simulink model "STEVE_ver28"  (R2022a)
settings: Solver=VariableStepAuto  StartTime=0.0  StopTime=Stop_Time  FixedStep=0.000001  RelTol=1e-5
values from neighbouring files (symbols this model uses):
  Bed_ave_OD = (1+Bed_ins_OD)/2    (= 1.667)    [STEVE_initialization.m]    (also in STEVE_running.m = (1+Bed_ins_OD)/2; STEVE_v4_C1Demo_2023_Nominal.m)
  Bed_ins_OD = 2.334    [STEVE_initialization.m]    (also in STEVE_v4_C1Demo_2023_Nominal.m)
  Bed_thickness = 0.049    [STEVE_initialization.m]    (also in STEVE_v4_C1Demo_2023_Nominal.m)
  Belimo_Cv = 16    [STEVE_initialization.m]    (also in STEVE_v4_C1Demo_2023_Nominal.m)
  flow_rate = 8    [STEVE_initialization.m]    (also in STEVE_v4_C1Demo_2023_Nominal.m)
  Heat_ads = 40000    [STEVE_initialization.m]    (also in STEVE_v4_C1Demo_2023_Nominal.m)
  Heater_output = 85.3    [STEVE_initialization.m]    (also in STEVE_v4_C1Demo_2023_Nominal.m)
  L = 0.508    [STEVE_initialization.m]    (also in STEVE_v4_C1Demo_2023_Nominal.m)
  L_inch = L*39.3701    (= 20.0000108)    [STEVE_initialization.m]    (also in STEVE_v4_C1Demo_2023_Nominal.m)
  max_temp = 200+273.15    (= 473.15)    [STEVE_initialization.m]    (also in STEVE_v4_C1Demo_2023_Nominal.m)
  mesh_size = 15    [STEVE_initialization.m]    (also in STEVE_v4_C1Demo_2023_Nominal.m)
  Pipe_ave_HD = (pipe_HD+0.5)/2    (= 0.465)    [STEVE_initialization.m]    (also in STEVE_running.m = (pipe_HD+0.5)/2; STEVE_v4_C1Demo_2023_Nominal.m)
  pipe_HD = 0.43    [STEVE_initialization.m]    (also in STEVE_v4_C1Demo_2023_Nominal.m)
  Ramp_rate = 0.0833    [STEVE_initialization.m]    (also in STEVE_v4_C1Demo_2023_Nominal.m)
  room_pressure = 13.3    [STEVE_initialization.m]    (also in STEVE_v4_C1Demo_2023_Nominal.m)
  t_Total = Adsorption_time + FlowStop_time + Valve_close_Time + Select_valve_close_Time + Pump_down_time + Desorption_time + SelectValve_open_Time + Valve_open_Time    (= 9635)    [STEVE_initialization.m]    (also in STEVE_running.m = Adsorption_time + FlowStop_time + Valve_close_Time + Select_; STEVE_v4_C1Demo_2023_Nominal.m)
libraries: fl_lib x229, nesl_utility x75, slpidlib x2
(part 2 of 5)

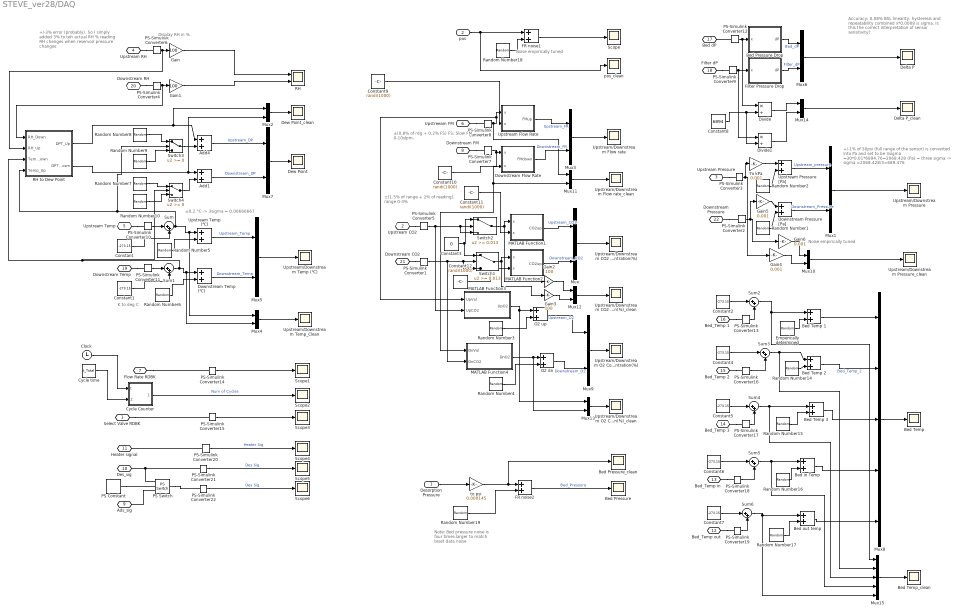
== system STEVE_ver28/DAQ ==
  note: Note: Bed pressure noise is four times larger to match teset data noise
  note: ±(1.5% of range + 2% of reading), range 0-3%
  note: ±0.2 °C -> 3sigma = 0.06666667
  note: ±(0.8% of rdg + 0.2% FS)
      | FS: Slow FM 0-10slpm,
  note: Accuracy: 0.08% BSL linearity, hysteresis and repeatability combined
      |
      | x*0.0008 is sigma. Is this the correct interpretation of sensor sensitivity?
  note: +/-1% of 30psi (full range of the sensor) is converted into Pa and set to be 3sigma
      | =30*0.01*6894.76=2068.428 (Pa) = three sigma  -> sigma =2068.428/3=689.476
  note: +/-3% error (probably). So I simply added 3% to teh actual RH % reading
      | RH chenges when reservoir pressure changes
  note: Display RH in %
  note: K to deg C
  note: Noise empirically tuned
  note: Noise empirically tuned
  Desorption Pressure : Inport
  pos : Inport  Port=2
  Add1 : Sum
  Add4 : Sum
  Bed Pressure : Scope
  Bed Pressure Drop : MATLAB Function  TreatAsAtomicUnit=on
  Bed Pressure_clean : Scope
  Bed Temp : Scope
  Bed Temp 1 : Sum
  Bed Temp 2 : Sum
  Bed Temp 3 : Sum
  Bed Temp_clean : Scope
  Bed in Temp : Sum
  Bed out temp : Sum
  Clock : Clock
  Constant{,1..2,4..7} (7 alike) : Constant  Value=-273.15
  Constant{9..12} (4 alike) : Constant  Value=randi(1000)
  Constant3 : Constant  Value=0
  Constant8 : Constant  Value=6894
  Cycle Counter : MATLAB Function  TreatAsAtomicUnit=on
  Cycle time : Constant  Value=t_Total
  Delta P : Scope
  Delta P_clean : Scope
  Dew Point : Scope
  Dew Point_clean : Scope
  Divide : Product  Inputs=*/
  Divide1 : Product  Inputs=*/
  Downstream Pressure [Pa] : Sum
  Downstream Temp (℃) : Sum
  Downstream Flow Rate : MATLAB Function  TreatAsAtomicUnit=on
  Emperically determined : RandomNumber  Variance=0.0197^2  Seed=randi(1000)  SampleTime=1  VectorParams1D=off
  FR noise1 : Sum
  FR noise2 : Sum
  Filter Pressure Drop : MATLAB Function  TreatAsAtomicUnit=on
  Gain{,1..3} (4 alike) : Gain  Gain=100
  Gain4 : Gain  Gain=0.001
  Gain5 : Gain  Gain=0.001
  Gain6 : Gain  Gain=0.001
  MATLAB Function1 : MATLAB Function  TreatAsAtomicUnit=on
  MATLAB Function2 : MATLAB Function  TreatAsAtomicUnit=on
  MATLAB Function3 : MATLAB Function  TreatAsAtomicUnit=on
  MATLAB Function4 : MATLAB Function  TreatAsAtomicUnit=on
  Mux{,1..7,9..14} (14 alike) : Mux  Inputs=2
  Mux15 : Mux  Inputs=5
  Mux8 : Mux  Inputs=5
  O2 dn : Sum
  O2 up : Sum
  PS Constant : fl_lib/Physical Signals/Sources/PS Constant  constant=0
      settings: SourceProductBaseCode=PW,SS,VE
  PS Switch : fl_lib/Physical Signals/Nonlinear Operators/PS Switch  Threshold=1
      settings: SourceProductBaseCode=PW,SS,VE  InternalSimscapePortConfiguration="{\"Bottom\":[],\"Left\":[{\"id\":\"I1\",\"label\":\"\",\"type\":\"input\"},{\"id\":\"I2\",\"label\":\"\",\"type\":\"input\"},{\"id\":\"I3\",\"label\":\"\",\"type\":\"input\"}],\"Right\":[{\"id\":\"O\",\"label\":\"\",\"type\":\"output\"}],\"Top\":[]}"
  PS-Simulink Converter{1,4..6,14..15,20..22} (9 alike) : nesl_utility/PS-Simulink Converter  PhysicalDomain=network_engine_domain  SubClassName=ps_output  LeftPortType=input  RightPortType=output  PseudoPeriodic=off  Frequencies=[]  VectorFormat=1-D array  Unit=inherit  AffineConversion=off
      settings: SourceProductBaseCode=SS,PW,VE
  PS-Simulink Converter{10..11,13,16..19} (7 alike) : nesl_utility/PS-Simulink Converter  PhysicalDomain=network_engine_domain  SubClassName=ps_output  LeftPortType=input  RightPortType=output  PseudoPeriodic=off  Frequencies=[]  VectorFormat=1-D array  Unit=K  AffineConversion=off
      settings: SourceProductBaseCode=SS,PW,VE
  PS-Simulink Converter{2..3,9,12} (4 alike) : nesl_utility/PS-Simulink Converter  PhysicalDomain=network_engine_domain  SubClassName=ps_output  LeftPortType=input  RightPortType=output  PseudoPeriodic=off  Frequencies=[]  VectorFormat=1-D array  Unit=Pa  AffineConversion=off
      settings: SourceProductBaseCode=SS,PW,VE
  PS-Simulink Converter7 : nesl_utility/PS-Simulink Converter  PhysicalDomain=network_engine_domain  SubClassName=ps_output  LeftPortType=input  RightPortType=output  PseudoPeriodic=off  Frequencies=[]  VectorFormat=1-D array  Unit=lpm  AffineConversion=off
      settings: SourceProductBaseCode=SS,PW,VE
  PS-Simulink Converter8 : nesl_utility/PS-Simulink Converter  PhysicalDomain=network_engine_domain  SubClassName=ps_output  LeftPortType=input  RightPortType=output  PseudoPeriodic=off  Frequencies=[]  VectorFormat=1-D array  Unit=lpm  AffineConversion=off
      settings: SourceProductBaseCode=SS,PW,VE
  RH : Scope  NumInputPorts=2
  RH to Dew Point : MATLAB Function  TreatAsAtomicUnit=on
  Random Number1 : RandomNumber  Variance=0.0068  Seed=randi(1000)  SampleTime=1  VectorParams1D=off
  Random Number10 : RandomNumber  Variance=(4/3)^2  Seed=randi(1000)  SampleTime=1  VectorParams1D=off
  Random Number{14..17} (4 alike) : RandomNumber  Variance=0.0197^2  Seed=randi(1000)  SampleTime=1  VectorParams1D=off
  Random Number18 : RandomNumber  Variance=0.0542  Seed=randi(1000)  SampleTime=1  VectorParams1D=off
  Random Number19 : RandomNumber  Variance=0.0326^2  Seed=randi(1000)  SampleTime=1  VectorParams1D=off
  Random Number2 : RandomNumber  Variance=0.0068  Seed=randi(1000)  SampleTime=1  VectorParams1D=off
  Random Number3 : RandomNumber  Variance=0.0175^2  Seed=randi(1000)  SampleTime=1  VectorParams1D=off
  Random Number4 : RandomNumber  Variance=0.0175^2  Seed=randi(1000)  SampleTime=1  VectorParams1D=off
  Random Number5 : RandomNumber  Variance=(0.06666667/3)^2  Seed=randi(1000)  SampleTime=1  VectorParams1D=off
  Random Number6 : RandomNumber  Variance=(0.06666667/3)^2  Seed=randi(1000)  SampleTime=1  VectorParams1D=off
  Random Number7 : RandomNumber  Variance=(2/3)^2  Seed=randi(1000)  SampleTime=1  VectorParams1D=off
  Random Number8 : RandomNumber  Variance=(2/3)^2  Seed=randi(1000)  SampleTime=1  VectorParams1D=off
  Random Number9 : RandomNumber  Variance=(4/3)^2  Seed=randi(1000)  SampleTime=1  VectorParams1D=off
  Scope{,1..6} (7 alike) : Scope
  Sum{,1..6} (7 alike) : Sum  Inputs=|++
  Switch1 : Switch  Threshold=0.013  SaturateOnIntegerOverflow=off  InputSameDT=off
  Switch2 : Switch  Threshold=0.013  SaturateOnIntegerOverflow=off  InputSameDT=off
  Switch3 : Switch  SaturateOnIntegerOverflow=off  InputSameDT=off
  Switch4 : Switch  SaturateOnIntegerOverflow=off  InputSameDT=off
  To kPa : Gain  Gain=0.001
  Upstream Pressure [Pa] : Sum
  Upstream Temp (℃) : Sum
  Upstream Flow Rate : MATLAB Function  TreatAsAtomicUnit=on
  Upstream/Downstream CO2 Concentration(%) : Scope
  Upstream/Downstream CO2 Concentration(%)_clean : Scope
  Upstream/Downstream Flow rate : Scope
  Upstream/Downstream O2 Concentration(%) : Scope
  Upstream/Downstream O2 Concentration(%)_clean : Scope
  Upstream/Downstream Pressure : Scope
  Upstream/Downstream Pressure_clean : Scope
  Upstream/Downstream Temp (℃) : Scope
  Upstream/Downstream Flow rate_clean : Scope
  Upstream/Downstream Temp_Clean : Scope
  pos_clean : Scope
  to psi : Gain  Gain=0.000145
  Select Valve RDBK : PMIOPort  Side=Left
  Upstream CO2 : PMIOPort  Port=2  Side=Left
  Upstream Pressure : PMIOPort  Port=3  Side=Left
  Upstream RH : PMIOPort  Port=4  Side=Left
  Upstream Temp : PMIOPort  Port=5  Side=Left
  Upstreeam FM : PMIOPort  Port=6  Side=Left
  Flow Rate RDBK : PMIOPort  Port=7  Side=Left
  Downstream FM : PMIOPort  Port=8  Side=Left
  Ads_sig : PMIOPort  Port=9  Side=Left
  Des_sig : PMIOPort  Port=10  Side=Left
  Heater signal : PMIOPort  Port=11  Side=Right
  Bed_Temp out : PMIOPort  Port=12  Side=Right
  Bed_Temp in : PMIOPort  Port=13  Side=Right
  Bed_Temp 3 : PMIOPort  Port=14  Side=Right
  Bed_Temp 2 : PMIOPort  Port=15  Side=Right
  Bed_Temp 1 : PMIOPort  Port=16  Side=Right
  Bed dP : PMIOPort  Port=17  Side=Right
  Filter dP : PMIOPort  Port=18  Side=Right
  Downstream Temp : PMIOPort  Port=19  Side=Right
  Downstream RH : PMIOPort  Port=20  Side=Right
  Downstream CO2 : PMIOPort  Port=21  Side=Right
  Downstream Pressure : PMIOPort  Port=22  Side=Right
  wires:
  Mux1/1 -> Upstream/Downstream Pressure/1
  Mux3/1 -> Upstream/Downstream Flow rate/1
  Mux5/1 -> Upstream/Downstream Temp (℃)/1
  Random Number1/1 -> Downstream Pressure [Pa]/2
  Random Number2/1 -> Upstream Pressure [Pa]/2
  PS-Simulink Converter6/1 -> RH to Dew Point/2(RH_Up), Gain/1
  PS-Simulink Converter4/1 -> RH to Dew Point/1(RH_Down), Gain1/1
  PS-Simulink Converter8/1 -> Mux11/1, MATLAB Function3/1(UpVol), Upstream Flow Rate/1(x)
  PS-Simulink Converter7/1 -> Mux11/2, MATLAB Function4/1(DnVol), Downstream Flow Rate/1(x)
  Downstream Flow Rate/1(FMdown) -> Mux3/2  "Downstream_FR"
  Upstream Flow Rate/1(FMup) -> Mux3/1  "Upstream_FR"
  Random Number5/1 -> Upstream Temp (℃)/2
  Upstream Temp (℃)/1 -> Mux5/1  "Upstream_Temp"
  Random Number6/1 -> Downstream Temp (℃)/2
  Downstream Temp (℃)/1 -> Mux5/2  "Downstream_Temp"
  PS-Simulink Converter10/1 -> Sum/1
  Constant/1 -> Sum/2
  Sum/1 -> Mux4/1, Upstream Temp (℃)/1, Switch3/2, RH to Dew Point/4(Temp_Up)
  Constant1/1 -> Sum1/2
  PS-Simulink Converter11/1 -> Sum1/1
  Sum1/1 -> Switch4/2, RH to Dew Point/3(Temp_Down), Mux4/2, Downstream Temp (℃)/1
  Filter Pressure Drop/1(dP) -> Mux6/2  "Filter_dP"
  PS-Simulink Converter12/1 -> Divide/1, Bed Pressure Drop/1(x)
  Bed Pressure Drop/1(dP) -> Mux6/1  "Bed_dP"
  Mux6/1 -> Delta P/1
  PS-Simulink Converter3/1 -> To kPa/1, Gain4/1
  PS-Simulink Converter2/1 -> Gain5/1, Gain6/1
  PS-Simulink Converter13/1 -> Sum2/2
  Constant2/1 -> Sum2/1
  PS-Simulink Converter5/1 -> MATLAB Function3/2(UpCO2), Switch2/3, Switch2/2
  Constant3/1 -> Switch2/1, Switch1/1
  PS-Simulink Converter1/1 -> MATLAB Function4/2(DnCO2), Switch1/3, Switch1/2
  Switch1/1 -> Gain3/1, MATLAB Function2/1(x)
  MATLAB Function2/1(CO2up) -> Mux/2  "Downstream_CO2"
  Switch2/1 -> Gain2/1, MATLAB Function1/1(x)
  MATLAB Function1/1(CO2up) -> Mux/1  "Upstream_CO2"
  Mux/1 -> Upstream/Downstream CO2 Concentration(%)/1
  RH to Dew Point/2(DPT_Down) -> Mux2/2, Add1/1
  Mux7/1 -> Dew Point/1
  RH to Dew Point/1(DPT_Up) -> Mux2/1, Add4/1
  Add1/1 -> Mux7/2  "Downstream_DP"
  Add4/1 -> Mux7/1  "Upstream_DP"
  Random Number8/1 -> Switch3/1
  Switch3/1 -> Add4/2
  Random Number9/1 -> Switch3/3
  Switch4/1 -> Add1/2
  Random Number7/1 -> Switch4/1
  Random Number10/1 -> Switch4/3
  Mux8/1 -> Bed Temp/1
  Constant4/1 -> Sum3/1
  PS-Simulink Converter16/1 -> Sum3/2
  Constant5/1 -> Sum4/1
  PS-Simulink Converter17/1 -> Sum4/2
  Bed Temp 1/1 -> Mux8/1
  Emperically determined/1 -> Bed Temp 1/2
  Sum2/1 -> Mux15/1, Bed Temp 1/1
  Sum3/1 -> Bed Temp 2/1, Mux15/2
  Random Number14/1 -> Bed Temp 2/2
  Sum4/1 -> Bed Temp 3/1, Mux15/3
  Random Number15/1 -> Bed Temp 3/2
  Bed Temp 2/1 -> Mux8/2  "Bed_Temp_2"
  Bed Temp 3/1 -> Mux8/3
  Bed in Temp/1 -> Mux8/4
  Random Number16/1 -> Bed in Temp/2
  Sum5/1 -> Mux15/4, Bed in Temp/1
  Constant6/1 -> Sum5/1
  PS-Simulink Converter18/1 -> Sum5/2
  Constant7/1 -> Sum6/1
  PS-Simulink Converter19/1 -> Sum6/2
  Sum6/1 -> Bed out temp/1, Mux15/5
  Bed out temp/1 -> Mux8/5
  Random Number17/1 -> Bed out temp/2
  Random Number18/1 -> FR noise1/2
  pos/1 -> pos_clean/1, FR noise1/1
  Mux9/1 -> Upstream/Downstream O2 Concentration(%)/1
  Random Number19/1 -> FR noise2/2
  FR noise2/1 -> Bed Pressure/1  "Bed_Pressure"
  Random Number3/1 -> O2 up/2
  O2 up/1 -> Mux9/1  "Upstream_O2"
  MATLAB Function3/1(UpO2) -> Mux13/1, O2 up/1
  Random Number4/1 -> O2 dn/2
  MATLAB Function4/1(DnO2) -> Mux13/2, O2 dn/1
  O2 dn/1 -> Mux9/2  "Downstream_O2"
  PS-Simulink Converter20/1 -> Scope4/1  "Heater Sig"
  Clock/1 -> Cycle Counter/1(t)
  Cycle time/1 -> Cycle Counter/2(t_tot)
  Cycle Counter/1(cycle) -> Scope2/1  "Num of Cycles"
  PS-Simulink Converter21/1 -> Scope5/1  "Des Sig"
  Gain/1 -> RH/1
  Gain1/1 -> RH/2
  FR noise1/1 -> Scope/1
  PS-Simulink Converter14/1 -> Scope1/1
  PS-Simulink Converter15/1 -> Scope3/1
  PS-Simulink Converter22/1 -> Scope6/1  "Des Sig"
  Mux2/1 -> Dew Point_clean/1
  Mux4/1 -> Upstream/Downstream Temp_Clean/1
  Mux11/1 -> Upstream/Downstream Flow rate_clean/1
  Mux12/1 -> Upstream/Downstream CO2 Concentration(%)_clean/1
  Gain2/1 -> Mux12/1
  Gain3/1 -> Mux12/2
  Mux13/1 -> Upstream/Downstream O2 Concentration(%)_clean/1
  Mux14/1 -> Delta P_clean/1
  PS-Simulink Converter9/1 -> Filter Pressure Drop/1(x), Divide1/1
  Constant8/1 -> Divide1/2, Divide/2
  Divide/1 -> Mux14/1
  Divide1/1 -> Mux14/2
  Mux10/1 -> Upstream/Downstream Pressure_clean/1
  Mux15/1 -> Bed Temp_clean/1
  Desorption Pressure/1 -> to psi/1
  to psi/1 -> Bed Pressure_clean/1, FR noise2/1
  Upstream Pressure [Pa]/1 -> Mux1/1  "Upstream_pressure"
  Downstream Pressure [Pa]/1 -> Mux1/2  "Downstream_Pressure"
  Gain6/1 -> Mux10/1
  Gain4/1 -> Mux10/2
  To kPa/1 -> Upstream Pressure [Pa]/1
  Gain5/1 -> Downstream Pressure [Pa]/1
  Constant9/1 -> Upstream Flow Rate/2(s)
  Constant10/1 -> Downstream Flow Rate/2(s)
  Constant11/1 -> MATLAB Function1/2(s)
  Constant12/1 -> MATLAB Function2/2(s)
  connections:
  Downstream CO2/RConn1 -- PS-Simulink Converter1/LConn1
  Downstream RH/RConn1 -- PS-Simulink Converter4/LConn1
  Downstream Pressure/RConn1 -- PS-Simulink Converter2/LConn1
  Upstream CO2/RConn1 -- PS-Simulink Converter5/LConn1
  Upstream Pressure/RConn1 -- PS-Simulink Converter3/LConn1
  Upstream RH/RConn1 -- PS-Simulink Converter6/LConn1
  Downstream FM/RConn1 -- PS-Simulink Converter7/LConn1
  Upstreeam FM/RConn1 -- PS-Simulink Converter8/LConn1
  Upstream Temp/RConn1 -- PS-Simulink Converter10/LConn1
  Downstream Temp/RConn1 -- PS-Simulink Converter11/LConn1
  Filter dP/RConn1 -- PS-Simulink Converter9/LConn1
  PS-Simulink Converter12/LConn1 -- Bed dP/RConn1
  Bed_Temp 1/RConn1 -- PS-Simulink Converter13/LConn1
  Flow Rate RDBK/RConn1 -- PS-Simulink Converter14/LConn1
  Select Valve RDBK/RConn1 -- PS-Simulink Converter15/LConn1
  Bed_Temp 2/RConn1 -- PS-Simulink Converter16/LConn1
  Bed_Temp 3/RConn1 -- PS-Simulink Converter17/LConn1
  Bed_Temp in/RConn1 -- PS-Simulink Converter18/LConn1
  Bed_Temp out/RConn1 -- PS-Simulink Converter19/LConn1
  PS-Simulink Converter20/LConn1 -- Heater signal/RConn1
  PS-Simulink Converter21/LConn1 -- PS Switch/LConn1 -- Des_sig/RConn1
  PS Switch/RConn1 -- PS-Simulink Converter22/LConn1
  PS Switch/LConn3 -- Ads_sig/RConn1
  PS Constant/RConn1 -- PS Switch/LConn2

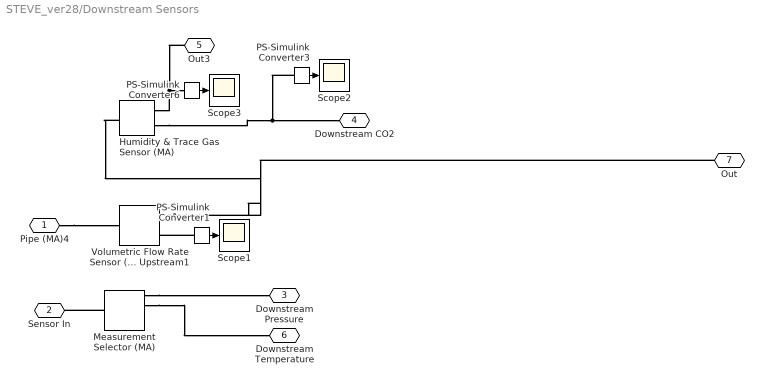
== system STEVE_ver28/Downstream Sensors ==
  Humidity & Trace Gas Sensor (MA) : fl_lib/Moist Air/Sensors/Humidity & Trace Gas Sensor (MA)  moisture_spec=foundation.enum.moisture_spec.relative_humidity  trace_gas_spec=foundation.enum.trace_gas_spec.mole_fraction
      settings: SourceProductBaseCode=PW,SS,VE  InternalSimscapePortConfiguration="{\"Bottom\":[],\"Left\":[{\"id\":\"A\",\"label\":\"A\",\"type\":\"foundation.moist_air.moist_air\"}],\"Right\":[{\"id\":\"W\",\"label\":\"W\",\"type\":\"output\"},{\"id\":\"G\",\"label\":\"G\",\"type\":\"output\"}],\"Top\":[]}"
  Measurement Selector (MA) : fl_lib/Moist Air/Sensors/Measurement Selector (MA)  moisture_spec=foundation.enum.moisture_spec.relative_humidity  trace_gas_spec=foundation.enum.trace_gas_spec.mass_fraction
      settings: SourceProductBaseCode=PW,SS,VE
  PS-Simulink Converter1 : nesl_utility/PS-Simulink Converter  PhysicalDomain=network_engine_domain  SubClassName=ps_output  LeftPortType=input  RightPortType=output  PseudoPeriodic=off  Frequencies=[]  VectorFormat=1-D array  Unit=lpm  AffineConversion=off
      settings: SourceProductBaseCode=SS,PW,VE
  PS-Simulink Converter3 : nesl_utility/PS-Simulink Converter  PhysicalDomain=network_engine_domain  SubClassName=ps_output  LeftPortType=input  RightPortType=output  PseudoPeriodic=off  Frequencies=[]  VectorFormat=1-D array  Unit=inherit  AffineConversion=off
      settings: SourceProductBaseCode=SS,PW,VE
  PS-Simulink Converter6 : nesl_utility/PS-Simulink Converter  PhysicalDomain=network_engine_domain  SubClassName=ps_output  LeftPortType=input  RightPortType=output  PseudoPeriodic=off  Frequencies=[]  VectorFormat=1-D array  Unit=kg/s  AffineConversion=off
      settings: SourceProductBaseCode=SS,PW,VE
  Scope1 : Scope
  Scope2 : Scope
  Scope3 : Scope
  Volumetric Flow Rate Sensor (MA) Upstream1 : fl_lib/Moist Air/Sensors/Volumetric Flow Rate Sensor (MA)  volumetric_flow_conditions=foundation.enum.volumetric_flow_conditions.actual  p_std=0.101325 MPa  T_std=20 degC  RH_std=0.65
      settings: SourceProductBaseCode=PW,SS,VE  InternalSimscapePortConfiguration="{\"Bottom\":[],\"Left\":[{\"id\":\"A\",\"label\":\"A\",\"type\":\"foundation.moist_air.moist_air\"}],\"Right\":[{\"id\":\"B\",\"label\":\"B\",\"type\":\"foundation.moist_air.moist_air\"},{\"id\":\"V\",\"label\":\"V\",\"type\":\"output\"}],\"Top\":[]}"
  Pipe (MA)4 : PMIOPort  Side=Left
  Sensor In : PMIOPort  Port=2  Side=Left
  Downstream Pressure : PMIOPort  Port=3  Side=Left
  Downstream CO2 : PMIOPort  Port=4  Side=Left
  Out3 : PMIOPort  Port=5  Side=Left
  Downstream Temperature : PMIOPort  Port=6  Side=Right
  Out : PMIOPort  Port=7  Side=Right
  wires:
  PS-Simulink Converter6/1 -> Scope3/1
  PS-Simulink Converter1/1 -> Scope1/1
  PS-Simulink Converter3/1 -> Scope2/1
  connections:
  Humidity & Trace Gas Sensor (MA)/RConn2 -- PS-Simulink Converter3/LConn1 -- Downstream CO2/RConn1
  Volumetric Flow Rate Sensor (MA) Upstream1/RConn1 -- Humidity & Trace Gas Sensor (MA)/LConn1 -- Out/RConn1
  Humidity & Trace Gas Sensor (MA)/RConn1 -- Out3/RConn1 -- PS-Simulink Converter6/LConn1
  PS-Simulink Converter1/LConn1 -- Volumetric Flow Rate Sensor (MA) Upstream1/RConn2
  Pipe (MA)4/RConn1 -- Volumetric Flow Rate Sensor (MA) Upstream1/LConn1
  Measurement Selector (MA)/RConn2 -- Downstream Temperature/RConn1
  Measurement Selector (MA)/LConn1 -- Sensor In/RConn1
  Measurement Selector (MA)/RConn1 -- Downstream Pressure/RConn1

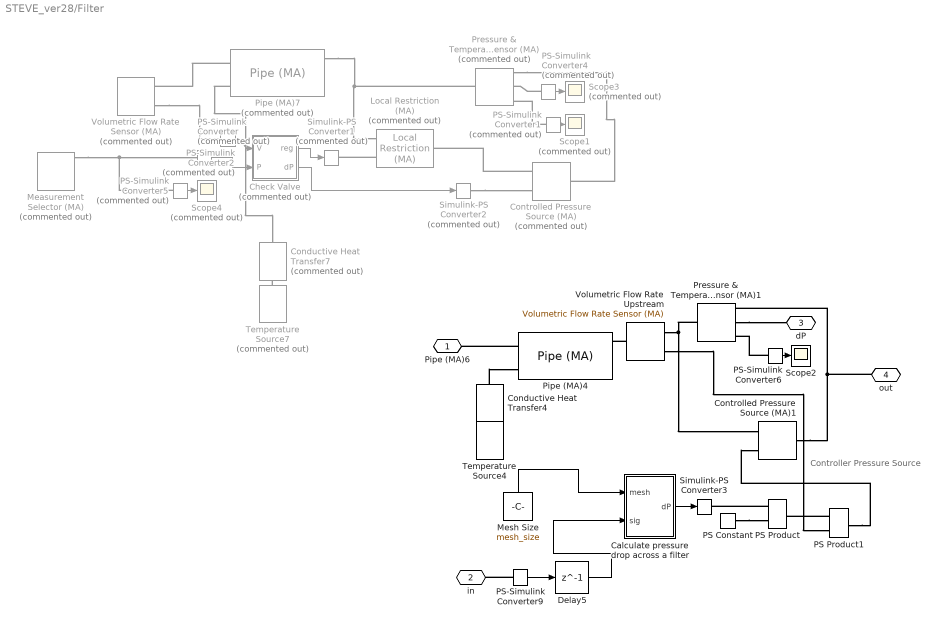
== system STEVE_ver28/Filter ==
  note: Controller Pressure Source
  Calculate pressure drop across a filter : MATLAB Function  TreatAsAtomicUnit=on
  Check Valve : MATLAB Function  Commented=on  TreatAsAtomicUnit=on
  Conductive Heat Transfer4 : fl_lib/Thermal/Thermal Elements/Conductive Heat Transfer  area=51.8 in^2  thickness=pipe_wall in  th_cond=pipe_tc W/(m*K)  T_specify=off  T_priority=None  T=0 K  T_nominal_specify=off  T_nominal_unit=K  T_nominal_value=1  Q_specify=off  Q_priority=None  Q=0 W  Q_nominal_specify=off  Q_nominal_unit=W  Q_nominal_value=1
      settings: SourceProductBaseCode=PW,SS,VE
  Conductive Heat Transfer7 : fl_lib/Thermal/Thermal Elements/Conductive Heat Transfer  Commented=on  area=51.8 in^2  thickness=0.048 in  th_cond=14.4 W/(m*K)  T_specify=off  T_priority=None  T=0 K  T_nominal_specify=off  T_nominal_unit=K  T_nominal_value=1  Q_specify=off  Q_priority=None  Q=0 W  Q_nominal_specify=off  Q_nominal_unit=W  Q_nominal_value=1
      settings: SourceProductBaseCode=PW,SS,VE
  Controlled Pressure Source (MA) : fl_lib/Moist Air/Sources/Controlled Pressure Source (MA)  Commented=on  power_spec=foundation.enum.power_spec.none  area_A=0.128 in^2  area_B=0.128 in^2
      settings: SourceProductBaseCode=PW,SS,VE  InternalSimscapePortConfiguration="{\"Bottom\":[],\"Left\":[{\"id\":\"A\",\"label\":\"A\",\"type\":\"foundation.moist_air.moist_air\"},{\"id\":\"P\",\"label\":\"P\",\"type\":\"input\"}],\"Right\":[{\"id\":\"B\",\"label\":\"B\",\"type\":\"foundation.moist_air.moist_air\"}],\"Top\":[]}"
  Controlled Pressure Source (MA)1 : fl_lib/Moist Air/Sources/Controlled Pressure Source (MA)  power_spec=foundation.enum.power_spec.none  area_A=(pi*pipe_HD^2)/4 in^2  area_B=(pi*pipe_HD^2)/4 in^2
      settings: SourceProductBaseCode=PW,SS,VE  InternalSimscapePortConfiguration="{\"Bottom\":[],\"Left\":[{\"id\":\"A\",\"label\":\"A\",\"type\":\"foundation.moist_air.moist_air\"},{\"id\":\"P\",\"label\":\"P\",\"type\":\"input\"}],\"Right\":[{\"id\":\"B\",\"label\":\"B\",\"type\":\"foundation.moist_air.moist_air\"}],\"Top\":[]}"
  Delay5 : Delay  DelayLength=1  InitialCondition=1
  Local Restriction (MA) : fl_lib/Moist Air/Elements/Local Restriction (MA)  Commented=on  restriction_type=foundation.enum.restriction_type.variable  restriction_area=0.001 m^2  min_area=1e-10 m^2  max_area=0.12799999 in^2  area=0.128 in^2  Cd=0.64  B_lam=0.999
      settings: SourceProductBaseCode=PW,SS,VE
  Measurement Selector (MA) : fl_lib/Moist Air/Sensors/Measurement Selector (MA)  Commented=on  moisture_spec=foundation.enum.moisture_spec.relative_humidity  trace_gas_spec=foundation.enum.trace_gas_spec.mass_fraction
      settings: SourceProductBaseCode=PW,SS,VE
  Mesh Size : Constant  Value=mesh_size
  PS Constant : fl_lib/Physical Signals/Sources/PS Constant  constant=60/(8*0.001) Pa/(m^3/s)
      settings: SourceProductBaseCode=PW,SS,VE
  PS Product : fl_lib/Physical Signals/Functions/PS Product
      settings: SourceProductBaseCode=PW,SS,VE
  PS Product1 : fl_lib/Physical Signals/Functions/PS Product
      settings: SourceProductBaseCode=PW,SS,VE
  PS-Simulink Converter : nesl_utility/PS-Simulink Converter  Commented=on  PhysicalDomain=network_engine_domain  SubClassName=ps_output  LeftPortType=input  RightPortType=output  PseudoPeriodic=off  Frequencies=[]  VectorFormat=1-D array  Unit=Pa  AffineConversion=off
      settings: SourceProductBaseCode=SS,PW,VE
  PS-Simulink Converter1 : nesl_utility/PS-Simulink Converter  Commented=on  PhysicalDomain=network_engine_domain  SubClassName=ps_output  LeftPortType=input  RightPortType=output  PseudoPeriodic=off  Frequencies=[]  VectorFormat=1-D array  Unit=inherit  AffineConversion=off
      settings: SourceProductBaseCode=SS,PW,VE
  PS-Simulink Converter2 : nesl_utility/PS-Simulink Converter  Commented=on  PhysicalDomain=network_engine_domain  SubClassName=ps_output  LeftPortType=input  RightPortType=output  PseudoPeriodic=off  Frequencies=[]  VectorFormat=1-D array  Unit=inherit  AffineConversion=off
      settings: SourceProductBaseCode=SS,PW,VE
  PS-Simulink Converter4 : nesl_utility/PS-Simulink Converter  Commented=on  PhysicalDomain=network_engine_domain  SubClassName=ps_output  LeftPortType=input  RightPortType=output  PseudoPeriodic=off  Frequencies=[]  VectorFormat=1-D array  Unit=Pa  AffineConversion=off
      settings: SourceProductBaseCode=SS,PW,VE
  PS-Simulink Converter5 : nesl_utility/PS-Simulink Converter  Commented=on  PhysicalDomain=network_engine_domain  SubClassName=ps_output  LeftPortType=input  RightPortType=output  PseudoPeriodic=off  Frequencies=[]  VectorFormat=1-D array  Unit=Pa  AffineConversion=off
      settings: SourceProductBaseCode=SS,PW,VE
  PS-Simulink Converter6 : nesl_utility/PS-Simulink Converter  PhysicalDomain=network_engine_domain  SubClassName=ps_output  LeftPortType=input  RightPortType=output  PseudoPeriodic=off  Frequencies=[]  VectorFormat=1-D array  Unit=inherit  AffineConversion=off
      settings: SourceProductBaseCode=SS,PW,VE
  PS-Simulink Converter9 : nesl_utility/PS-Simulink Converter  PhysicalDomain=network_engine_domain  SubClassName=ps_output  LeftPortType=input  RightPortType=output  PseudoPeriodic=off  Frequencies=[]  VectorFormat=1-D array  Unit=inherit  AffineConversion=off
      settings: SourceProductBaseCode=SS,PW,VE
  Pipe (MA)4 : fl_lib/Moist Air/Elements/Pipe (MA)  length=3 in  area=(pi*pipe_HD^2)/4 in^2  Dh=pipe_HD in  length_add=0.1 m  roughness=roughness m  Re_lam=2000  Re_tur=4000  shape_factor=64  Nu_lam=3.66  RH_ws=1  time_constant=1e-3 s  moisture_trace_gas_source=foundation.enum.moisture_trace_gas_source.none  moisture_source_spec=foundation.enum.moisture_source_spec.vapor  moisture_mass_flow=0 kg/s  moisture_temperature_spec=foundation.enum.temperature_spec.atmospheric  moisture_temperature=293.15 K  trace_gas_mass_flow=0 kg/s  trace_gas_temperature_spec=foundation.enum.temperature_spec.atmospheric  trace_gas_temperature=293.15 K  p_I_specify=off  p_I_priority=High  p_I=0.101325 MPa  p_I_nominal_specify=off  p_I_nominal_unit=MPa  p_I_nominal_value=1  T_I_specify=off  T_I_priority=High  T_I=293.15 K  T_I_nominal_specify=off  T_I_nominal_unit=K  T_I_nominal_value=1  RH_I_specify=off  RH_I_priority=High  RH_I=0  RH_I_nominal_specify=off  RH_I_nominal_unit=1  RH_I_nominal_value=1  x_w_I_specify=off  x_w_I_priority=None  x_w_I=0  x_w_I_nominal_specify=off  x_w_I_nominal_unit=1  x_w_I_nominal_value=1  y_w_I_specify=off  y_w_I_priority=None  y_w_I=0  y_w_I_nominal_specify=off  y_w_I_nominal_unit=1  y_w_I_nominal_value=1  HR_I_specify=off  HR_I_priority=None  HR_I=0  HR_I_nominal_specify=off  HR_I_nominal_unit=1  HR_I_nominal_value=1  x_g_I_specify=off  x_g_I_priority=High  x_g_I=0  x_g_I_nominal_specify=off  x_g_I_nominal_unit=1  x_g_I_nominal_value=1  y_g_I_specify=off  y_g_I_priority=None  y_g_I=0  y_g_I_nominal_specify=off  y_g_I_nominal_unit=1  y_g_I_nominal_value=1
      settings: SourceProductBaseCode=PW,SS,VE
  Pipe (MA)7 : fl_lib/Moist Air/Elements/Pipe (MA)  Commented=on  length=3 in  area=0.128 in^2  Dh=0.4035 in  length_add=0.1 m  roughness=15e-6 m  Re_lam=2000  Re_tur=4000  shape_factor=64  Nu_lam=3.66  RH_ws=1  time_constant=1e-3 s  moisture_trace_gas_source=foundation.enum.moisture_trace_gas_source.none  moisture_source_spec=foundation.enum.moisture_source_spec.vapor  moisture_mass_flow=0 kg/s  moisture_temperature_spec=foundation.enum.temperature_spec.atmospheric  moisture_temperature=293.15 K  trace_gas_mass_flow=0 kg/s  trace_gas_temperature_spec=foundation.enum.temperature_spec.atmospheric  trace_gas_temperature=293.15 K  p_I_specify=off  p_I_priority=High  p_I=0.101325 MPa  p_I_nominal_specify=off  p_I_nominal_unit=MPa  p_I_nominal_value=1  T_I_specify=off  T_I_priority=High  T_I=293.15 K  T_I_nominal_specify=off  T_I_nominal_unit=K  T_I_nominal_value=1  RH_I_specify=off  RH_I_priority=High  RH_I=0  RH_I_nominal_specify=off  RH_I_nominal_unit=1  RH_I_nominal_value=1  x_w_I_specify=off  x_w_I_priority=None  x_w_I=0  x_w_I_nominal_specify=off  x_w_I_nominal_unit=1  x_w_I_nominal_value=1  y_w_I_specify=off  y_w_I_priority=None  y_w_I=0  y_w_I_nominal_specify=off  y_w_I_nominal_unit=1  y_w_I_nominal_value=1  HR_I_specify=off  HR_I_priority=None  HR_I=0  HR_I_nominal_specify=off  HR_I_nominal_unit=1  HR_I_nominal_value=1  x_g_I_specify=off  x_g_I_priority=High  x_g_I=0  x_g_I_nominal_specify=off  x_g_I_nominal_unit=1  x_g_I_nominal_value=1  y_g_I_specify=off  y_g_I_priority=None  y_g_I=0  y_g_I_nominal_specify=off  y_g_I_nominal_unit=1  y_g_I_nominal_value=1
      settings: SourceProductBaseCode=PW,SS,VE
  Pressure & Temperature Sensor (MA) : fl_lib/Moist Air/Sensors/Pressure & Temperature Sensor (MA)  Commented=on
      settings: SourceProductBaseCode=PW,SS,VE  InternalSimscapePortConfiguration="{\"Bottom\":[],\"Left\":[{\"id\":\"A\",\"label\":\"A\",\"type\":\"foundation.moist_air.moist_air\"}],\"Right\":[{\"id\":\"B\",\"label\":\"B\",\"type\":\"foundation.moist_air.moist_air\"},{\"id\":\"P\",\"label\":\"P\",\"type\":\"output\"},{\"id\":\"T\",\"label\":\"T\",\"type\":\"output\"}],\"Top\":[]}"
  Pressure & Temperature Sensor (MA)1 : fl_lib/Moist Air/Sensors/Pressure & Temperature Sensor (MA)
      settings: SourceProductBaseCode=PW,SS,VE  InternalSimscapePortConfiguration="{\"Bottom\":[],\"Left\":[{\"id\":\"A\",\"label\":\"A\",\"type\":\"foundation.moist_air.moist_air\"}],\"Right\":[{\"id\":\"B\",\"label\":\"B\",\"type\":\"foundation.moist_air.moist_air\"},{\"id\":\"P\",\"label\":\"P\",\"type\":\"output\"},{\"id\":\"T\",\"label\":\"T\",\"type\":\"output\"}],\"Top\":[]}"
  Scope1 : Scope  Commented=on
  Scope2 : Scope
  Scope3 : Scope  Commented=on
  Scope4 : Scope  Commented=on
  Simulink-PS Converter1 : nesl_utility/Simulink-PS Converter  Commented=on  PhysicalDomain=network_engine_domain  SubClassName=ps_input  LeftPortType=input  RightPortType=output  PseudoPeriodic=off  Frequencies=[]  NoiseDistribution=none  NoiseParameters=[]  Unit=in^2  AffineConversion=off  FilteringAndDerivatives=provide  SimscapeFilterOrder=1  InputFilterTimeConstant=0.001  UdotUserProvided=0
      settings: SourceProductBaseCode=SS,PW,VE
  Simulink-PS Converter2 : nesl_utility/Simulink-PS Converter  Commented=on  PhysicalDomain=network_engine_domain  SubClassName=ps_input  LeftPortType=input  RightPortType=output  PseudoPeriodic=off  Frequencies=[]  NoiseDistribution=none  NoiseParameters=[]  Unit=Pa  AffineConversion=off  FilteringAndDerivatives=provide  SimscapeFilterOrder=1  InputFilterTimeConstant=0.001  UdotUserProvided=0
      settings: SourceProductBaseCode=SS,PW,VE
  Simulink-PS Converter3 : nesl_utility/Simulink-PS Converter  PhysicalDomain=network_engine_domain  SubClassName=ps_input  LeftPortType=input  RightPortType=output  PseudoPeriodic=off  Frequencies=[]  NoiseDistribution=none  NoiseParameters=[]  Unit=1  AffineConversion=off  FilteringAndDerivatives=provide  SimscapeFilterOrder=1  InputFilterTimeConstant=0.001  UdotUserProvided=0
      settings: SourceProductBaseCode=SS,PW,VE
  Temperature Source4 : fl_lib/Thermal/Thermal Sources/Temperature Source  temperature=room_temp K
      settings: SourceProductBaseCode=PW,SS,VE
  Temperature Source7 : fl_lib/Thermal/Thermal Sources/Temperature Source  Commented=on  temperature=293.15 K
      settings: SourceProductBaseCode=PW,SS,VE
  Volumetric Flow Rate Upstream : fl_lib/Moist Air/Sensors/Volumetric Flow Rate Sensor (MA)  volumetric_flow_conditions=foundation.enum.volumetric_flow_conditions.actual  p_std=0.101325 MPa  T_std=20 degC  RH_std=0.65
      settings: SourceProductBaseCode=PW,SS,VE  InternalSimscapePortConfiguration="{\"Bottom\":[],\"Left\":[{\"id\":\"A\",\"label\":\"A\",\"type\":\"foundation.moist_air.moist_air\"}],\"Right\":[{\"id\":\"B\",\"label\":\"B\",\"type\":\"foundation.moist_air.moist_air\"},{\"id\":\"V\",\"label\":\"V\",\"type\":\"output\"}],\"Top\":[]}"
  Volumetric Flow Rate Sensor (MA) : fl_lib/Moist Air/Sensors/Volumetric Flow Rate Sensor (MA)  Commented=on  volumetric_flow_conditions=foundation.enum.volumetric_flow_conditions.actual  p_std=0.101325 MPa  T_std=20 degC  RH_std=0.65
      settings: SourceProductBaseCode=PW,SS,VE  InternalSimscapePortConfiguration="{\"Bottom\":[],\"Left\":[{\"id\":\"A\",\"label\":\"A\",\"type\":\"foundation.moist_air.moist_air\"}],\"Right\":[{\"id\":\"B\",\"label\":\"B\",\"type\":\"foundation.moist_air.moist_air\"},{\"id\":\"V\",\"label\":\"V\",\"type\":\"output\"}],\"Top\":[]}"
  Pipe (MA)6 : PMIOPort  Side=Left
  in : PMIOPort  Port=2  Side=Left
  dP : PMIOPort  Port=3  Side=Left
  out : PMIOPort  Port=4  Side=Right
  wires:
  PS-Simulink Converter4/1 -> Scope3/1
  Check Valve/1(reg) -> Simulink-PS Converter1/1
  PS-Simulink Converter/1 -> Check Valve/2(P)
  PS-Simulink Converter1/1 -> Scope1/1
  PS-Simulink Converter2/1 -> Check Valve/1(V)
  Check Valve/2(dP) -> Simulink-PS Converter2/1
  PS-Simulink Converter5/1 -> Scope4/1
  PS-Simulink Converter6/1 -> Scope2/1
  Calculate pressure drop across a filter/1(dP) -> Simulink-PS Converter3/1
  Mesh Size/1 -> Calculate pressure drop across a filter/1(mesh)
  PS-Simulink Converter9/1 -> Delay5/1
  Delay5/1 -> Calculate pressure drop across a filter/2(sig)
  connections:
  Pressure & Temperature Sensor (MA)/RConn1 -- Controlled Pressure Source (MA)/RConn1
  PS-Simulink Converter1/LConn1 -- Pressure & Temperature Sensor (MA)/RConn3
  Local Restriction (MA)/LConn2 -- Simulink-PS Converter1/RConn1
  PS-Simulink Converter4/LConn1 -- Pressure & Temperature Sensor (MA)/RConn2
  Pressure & Temperature Sensor (MA)/LConn1 -- Pipe (MA)7/RConn1 -- Local Restriction (MA)/LConn1
  Controlled Pressure Source (MA)/LConn1 -- Local Restriction (MA)/RConn1
  Volumetric Flow Rate Sensor (MA)/RConn2 -- PS-Simulink Converter2/LConn1
  Simulink-PS Converter2/RConn1 -- Controlled Pressure Source (MA)/LConn2
  Measurement Selector (MA)/RConn1 -- PS-Simulink Converter5/LConn1 -- PS-Simulink Converter/LConn1
  Controlled Pressure Source (MA)1/RConn1 -- out/RConn1 -- Pressure & Temperature Sensor (MA)1/RConn1
  Pressure & Temperature Sensor (MA)1/LConn1 -- Volumetric Flow Rate Upstream/RConn1 -- Controlled Pressure Source (MA)1/LConn1
  Pressure & Temperature Sensor (MA)1/RConn2 -- dP/RConn1
  Temperature Source4/LConn1 -- Conductive Heat Transfer4/RConn1
  PS-Simulink Converter6/LConn1 -- Pressure & Temperature Sensor (MA)1/RConn3
  Conductive Heat Transfer4/LConn1 -- Pipe (MA)4/LConn2
  Pipe (MA)7/LConn1 -- Volumetric Flow Rate Sensor (MA)/RConn1
  Temperature Source7/LConn1 -- Conductive Heat Transfer7/RConn1
  Pipe (MA)7/LConn2 -- Conductive Heat Transfer7/LConn1
  Pipe (MA)4/LConn1 -- Pipe (MA)6/RConn1
  Volumetric Flow Rate Upstream/LConn1 -- Pipe (MA)4/RConn1
  Volumetric Flow Rate Upstream/RConn2 -- PS Product1/LConn2
  PS Product/LConn1 -- Simulink-PS Converter3/RConn1
  PS Constant/RConn1 -- PS Product/LConn2
  PS Product1/LConn1 -- PS Product/RConn1
  PS Product1/RConn1 -- Controlled Pressure Source (MA)1/LConn2
  PS-Simulink Converter9/LConn1 -- in/RConn1

== system STEVE_ver28/Flow Meter ==
  Volumetric Flow Rate Sensor (MA) Downstream : fl_lib/Moist Air/Sensors/Volumetric Flow Rate Sensor (MA)  volumetric_flow_conditions=foundation.enum.volumetric_flow_conditions.actual  p_std=0.101325 MPa  T_std=20 degC  RH_std=0.65
      settings: SourceProductBaseCode=PW,SS,VE  InternalSimscapePortConfiguration="{\"Bottom\":[],\"Left\":[{\"id\":\"A\",\"label\":\"A\",\"type\":\"foundation.moist_air.moist_air\"}],\"Right\":[{\"id\":\"B\",\"label\":\"B\",\"type\":\"foundation.moist_air.moist_air\"},{\"id\":\"V\",\"label\":\"V\",\"type\":\"output\"}],\"Top\":[]}"
  In : PMIOPort  Side=Left
  Downstream Flow Rate : PMIOPort  Port=2  Side=Left
  Out : PMIOPort  Port=3  Side=Right
  connections:
  Volumetric Flow Rate Sensor (MA) Downstream/RConn1 -- Out/RConn1
  In/RConn1 -- Volumetric Flow Rate Sensor (MA) Downstream/LConn1
  Volumetric Flow Rate Sensor (MA) Downstream/RConn2 -- Downstream Flow Rate/RConn1

== system STEVE_ver28/Flow meter ==
  Volumetric Flow Rate Sensor (MA) Upstream : fl_lib/Moist Air/Sensors/Volumetric Flow Rate Sensor (MA)  volumetric_flow_conditions=foundation.enum.volumetric_flow_conditions.actual  p_std=0.101325 MPa  T_std=20 degC  RH_std=0.65
      settings: SourceProductBaseCode=PW,SS,VE  InternalSimscapePortConfiguration="{\"Bottom\":[],\"Left\":[{\"id\":\"A\",\"label\":\"A\",\"type\":\"foundation.moist_air.moist_air\"}],\"Right\":[{\"id\":\"B\",\"label\":\"B\",\"type\":\"foundation.moist_air.moist_air\"},{\"id\":\"V\",\"label\":\"V\",\"type\":\"output\"}],\"Top\":[]}"
  Out : PMIOPort  Side=Right
  In : PMIOPort  Port=2  Side=Left
  Upstream Flow Rate : PMIOPort  Port=3  Side=Right
  connections:
  In/RConn1 -- Volumetric Flow Rate Sensor (MA) Upstream/LConn1
  Upstream Flow Rate/RConn1 -- Volumetric Flow Rate Sensor (MA) Upstream/RConn2
  Volumetric Flow Rate Sensor (MA) Upstream/RConn1 -- Out/RConn1

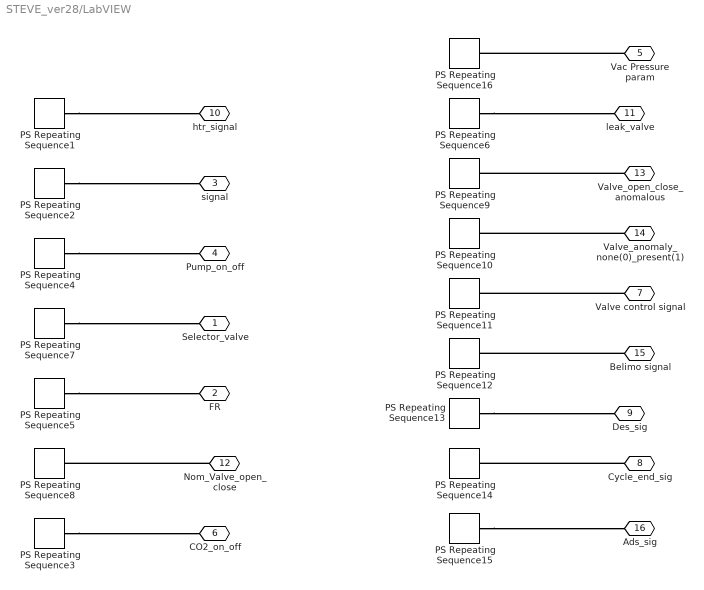
== system STEVE_ver28/LabVIEW ==
  PS Repeating Sequence1 : fl_lib/Physical Signals/Sources/PS Repeating Sequence  y_init=0  offset=0 s  sig_type=1  durations=Timing s  y_start=htr_signal_st  y_end=htr_signal_end
      settings: SourceProductBaseCode=PW,SS,VE  InternalSimscapePortConfiguration="{\"Bottom\":[],\"Left\":[],\"Right\":[{\"id\":\"Y\",\"label\":\"Y\",\"type\":\"output\"}],\"Top\":[]}"
  PS Repeating Sequence10 : fl_lib/Physical Signals/Sources/PS Repeating Sequence  y_init=0  offset=0 s  sig_type=1  durations=Anomaly_timing s  y_start=valve_anom_signal_st  y_end=valve_anom_signal_end
      settings: SourceProductBaseCode=PW,SS,VE  InternalSimscapePortConfiguration="{\"Bottom\":[],\"Left\":[],\"Right\":[{\"id\":\"Y\",\"label\":\"Y\",\"type\":\"output\"}],\"Top\":[]}"
  PS Repeating Sequence11 : fl_lib/Physical Signals/Sources/PS Repeating Sequence  y_init=0  offset=0 s  sig_type=1  durations=Timing s  y_start=valve_cont_sig  y_end=valve_cont_sig
      settings: SourceProductBaseCode=PW,SS,VE  InternalSimscapePortConfiguration="{\"Bottom\":[],\"Left\":[],\"Right\":[{\"id\":\"Y\",\"label\":\"Y\",\"type\":\"output\"}],\"Top\":[]}"
  PS Repeating Sequence12 : fl_lib/Physical Signals/Sources/PS Repeating Sequence  y_init=0  offset=0 s  sig_type=1  durations=Timing s  y_start=belimo_sig  y_end=belimo_sig
      settings: SourceProductBaseCode=PW,SS,VE  InternalSimscapePortConfiguration="{\"Bottom\":[],\"Left\":[],\"Right\":[{\"id\":\"Y\",\"label\":\"Y\",\"type\":\"output\"}],\"Top\":[]}"
  PS Repeating Sequence13 : fl_lib/Physical Signals/Sources/PS Repeating Sequence  y_init=1  offset=0 s  sig_type=1  durations=Timing s  y_start=Des_st  y_end=Des_end
      settings: SourceProductBaseCode=PW,SS,VE  InternalSimscapePortConfiguration="{\"Bottom\":[],\"Left\":[],\"Right\":[{\"id\":\"Y\",\"label\":\"Y\",\"type\":\"output\"}],\"Top\":[]}"
  PS Repeating Sequence14 : fl_lib/Physical Signals/Sources/PS Repeating Sequence  y_init=0  offset=0 s  sig_type=1  durations=Timing s  y_start=cycle_end_sig  y_end=cycle_end_sig
      settings: SourceProductBaseCode=PW,SS,VE  InternalSimscapePortConfiguration="{\"Bottom\":[],\"Left\":[],\"Right\":[{\"id\":\"Y\",\"label\":\"Y\",\"type\":\"output\"}],\"Top\":[]}"
  PS Repeating Sequence15 : fl_lib/Physical Signals/Sources/PS Repeating Sequence  y_init=0  offset=0 s  sig_type=1  durations=Timing s  y_start=Ads_st  y_end=Ads_end
      settings: SourceProductBaseCode=PW,SS,VE  InternalSimscapePortConfiguration="{\"Bottom\":[],\"Left\":[],\"Right\":[{\"id\":\"Y\",\"label\":\"Y\",\"type\":\"output\"}],\"Top\":[]}"
  PS Repeating Sequence16 : fl_lib/Physical Signals/Sources/PS Repeating Sequence  y_init=0  offset=0 s  sig_type=1  durations=Anomaly_timing s  y_start=vac_anom_st  y_end=vac_anom_end
      settings: SourceProductBaseCode=PW,SS,VE  InternalSimscapePortConfiguration="{\"Bottom\":[],\"Left\":[],\"Right\":[{\"id\":\"Y\",\"label\":\"Y\",\"type\":\"output\"}],\"Top\":[]}"
  PS Repeating Sequence2 : fl_lib/Physical Signals/Sources/PS Repeating Sequence  y_init=0  offset=0 s  sig_type=1  durations=Timing s  y_start=signal_st  y_end=signal_end
      settings: SourceProductBaseCode=PW,SS,VE  InternalSimscapePortConfiguration="{\"Bottom\":[],\"Left\":[],\"Right\":[{\"id\":\"Y\",\"label\":\"Y\",\"type\":\"output\"}],\"Top\":[]}"
  PS Repeating Sequence3 : fl_lib/Physical Signals/Sources/PS Repeating Sequence  y_init=1  offset=0 s  sig_type=1  durations=Timing s  y_start=CO2_st  y_end=CO2_end
      settings: SourceProductBaseCode=PW,SS,VE  InternalSimscapePortConfiguration="{\"Bottom\":[],\"Left\":[],\"Right\":[{\"id\":\"Y\",\"label\":\"Y\",\"type\":\"output\"}],\"Top\":[]}"
  PS Repeating Sequence4 : fl_lib/Physical Signals/Sources/PS Repeating Sequence  y_init=1e-10  offset=0 s  sig_type=1  durations=Timing s  y_start=Pump_on_off_st  y_end=Pump_on_off_end
      settings: SourceProductBaseCode=PW,SS,VE  InternalSimscapePortConfiguration="{\"Bottom\":[],\"Left\":[],\"Right\":[{\"id\":\"Y\",\"label\":\"Y\",\"type\":\"output\"}],\"Top\":[]}"
  PS Repeating Sequence5 : fl_lib/Physical Signals/Sources/PS Repeating Sequence  y_init=flow_rate*0.001/60  offset=0 s  sig_type=1  durations=Timing s  y_start=FR_st  y_end=FR_end
      settings: SourceProductBaseCode=PW,SS,VE  InternalSimscapePortConfiguration="{\"Bottom\":[],\"Left\":[],\"Right\":[{\"id\":\"Y\",\"label\":\"Y\",\"type\":\"output\"}],\"Top\":[]}"
  PS Repeating Sequence6 : fl_lib/Physical Signals/Sources/PS Repeating Sequence  y_init=1  offset=0 s  sig_type=1  durations=Anomaly_timing s  y_start=Leak_valve_deg_st  y_end=Leak_valve_deg_end
      settings: SourceProductBaseCode=PW,SS,VE  InternalSimscapePortConfiguration="{\"Bottom\":[],\"Left\":[],\"Right\":[{\"id\":\"Y\",\"label\":\"Y\",\"type\":\"output\"}],\"Top\":[]}"
  PS Repeating Sequence7 : fl_lib/Physical Signals/Sources/PS Repeating Sequence  y_init=(pi*(0.43-0.0001)^2)/4  offset=0 s  sig_type=1  durations=Timing s  y_start=Select_valve_st  y_end=Select_valve_end
      settings: SourceProductBaseCode=PW,SS,VE  InternalSimscapePortConfiguration="{\"Bottom\":[],\"Left\":[],\"Right\":[{\"id\":\"Y\",\"label\":\"Y\",\"type\":\"output\"}],\"Top\":[]}"
  PS Repeating Sequence8 : fl_lib/Physical Signals/Sources/PS Repeating Sequence  y_init=(pi*(0.43-0.0001)^2)/4  offset=0 s  sig_type=1  durations=Timing s  y_start=Valve_op_cl_st  y_end=Valve_op_cl_end
      settings: SourceProductBaseCode=PW,SS,VE  InternalSimscapePortConfiguration="{\"Bottom\":[],\"Left\":[],\"Right\":[{\"id\":\"Y\",\"label\":\"Y\",\"type\":\"output\"}],\"Top\":[]}"
  PS Repeating Sequence9 : fl_lib/Physical Signals/Sources/PS Repeating Sequence  y_init=(pi*(0.43-0.0001)^2)/4  offset=0 s  sig_type=1  durations=Timing s  y_start=Bad_Valve_op_cl_st  y_end=Bad_Valve_op_cl_end
      settings: SourceProductBaseCode=PW,SS,VE  InternalSimscapePortConfiguration="{\"Bottom\":[],\"Left\":[],\"Right\":[{\"id\":\"Y\",\"label\":\"Y\",\"type\":\"output\"}],\"Top\":[]}"
  Selector_valve : PMIOPort  Side=Left
  FR : PMIOPort  Port=2  Side=Left
  signal : PMIOPort  Port=3  Side=Left
  Pump_on_off : PMIOPort  Port=4  Side=Left
  Vac Pressure param : PMIOPort  Port=5  Side=Left
  CO2_on_off : PMIOPort  Port=6  Side=Right
  Valve control signal : PMIOPort  Port=7  Side=Right
  Cycle_end_sig : PMIOPort  Port=8  Side=Right
  Des_sig : PMIOPort  Port=9  Side=Right
  htr_signal : PMIOPort  Port=10  Side=Right
  leak_valve : PMIOPort  Port=11  Side=Right
  Nom_Valve_open_close : PMIOPort  Port=12  Side=Right
  Valve_open_close_anomalous : PMIOPort  Port=13  Side=Right
  Valve_anomaly_none(0)_present(1) : PMIOPort  Port=14  Side=Right
  Belimo signal : PMIOPort  Port=15  Side=Right
  Ads_sig : PMIOPort  Port=16  Side=Right
  connections:
  PS Repeating Sequence4/RConn1 -- Pump_on_off/RConn1
  PS Repeating Sequence7/RConn1 -- Selector_valve/RConn1
  PS Repeating Sequence5/RConn1 -- FR/RConn1
  Nom_Valve_open_close/RConn1 -- PS Repeating Sequence8/RConn1
  PS Repeating Sequence2/RConn1 -- signal/RConn1
  PS Repeating Sequence3/RConn1 -- CO2_on_off/RConn1
  PS Repeating Sequence1/RConn1 -- htr_signal/RConn1
  PS Repeating Sequence6/RConn1 -- leak_valve/RConn1
  Valve_open_close_anomalous/RConn1 -- PS Repeating Sequence9/RConn1
  Valve_anomaly_none(0)_present(1)/RConn1 -- PS Repeating Sequence10/RConn1
  Valve control signal/RConn1 -- PS Repeating Sequence11/RConn1
  Belimo signal/RConn1 -- PS Repeating Sequence12/RConn1
  PS Repeating Sequence13/RConn1 -- Des_sig/RConn1
  Cycle_end_sig/RConn1 -- PS Repeating Sequence14/RConn1
  PS Repeating Sequence15/RConn1 -- Ads_sig/RConn1
  Vac Pressure param/RConn1 -- PS Repeating Sequence16/RConn1

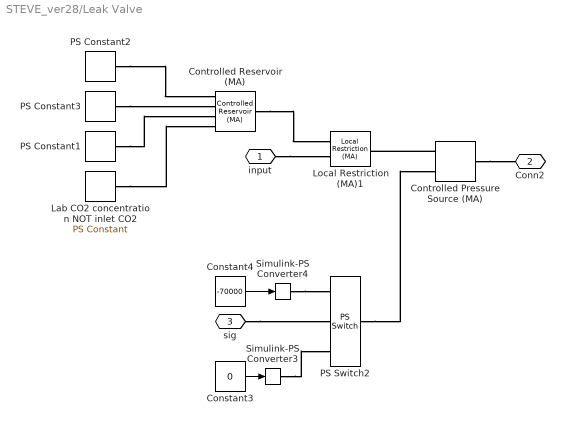
== system STEVE_ver28/Leak Valve ==
  Constant3 : Constant  Value=0
  Constant4 : Constant  Value=-70000
  Controlled Pressure Source (MA) : fl_lib/Moist Air/Sources/Controlled Pressure Source (MA)  power_spec=foundation.enum.power_spec.isentropic  area_A=(pi*pipe_HD^2)/4 in^2  area_B=(pi*pipe_HD^2)/4 in^2
      settings: SourceProductBaseCode=PW,SS,VE  InternalSimscapePortConfiguration="{\"Bottom\":[],\"Left\":[{\"id\":\"A\",\"label\":\"A\",\"type\":\"foundation.moist_air.moist_air\"},{\"id\":\"P\",\"label\":\"P\",\"type\":\"input\"}],\"Right\":[{\"id\":\"B\",\"label\":\"B\",\"type\":\"foundation.moist_air.moist_air\"}],\"Top\":[]}"
  Controlled Reservoir (MA) : fl_lib/Moist Air/Elements/Controlled Reservoir (MA)  moisture_spec=foundation.enum.moisture_spec.relative_humidity  trace_gas_spec=foundation.enum.trace_gas_spec.mass_fraction  RH_ws=1  area_A=(pi*pipe_HD^2)/4 in^2  input_error_spec=foundation.enum.input_range_error.warn
      settings: SourceProductBaseCode=PW,SS,VE  InternalSimscapePortConfiguration="{\"Bottom\":[],\"Left\":[{\"id\":\"A\",\"label\":\"A\",\"type\":\"foundation.moist_air.moist_air\"}],\"Right\":[{\"id\":\"T\",\"label\":\"T\",\"type\":\"input\"},{\"id\":\"P\",\"label\":\"P\",\"type\":\"input\"},{\"id\":\"W\",\"label\":\"W\",\"type\":\"input\"},{\"id\":\"G\",\"label\":\"G\",\"type\":\"input\"}],\"Top\":[]}"
  Lab CO2 concentration NOT inlet CO2 : fl_lib/Physical Signals/Sources/PS Constant  constant=0.0004
      settings: SourceProductBaseCode=PW,SS,VE
  Local Restriction (MA)1 : fl_lib/Moist Air/Elements/Local Restriction (MA)  restriction_type=foundation.enum.restriction_type.variable  restriction_area=0.001 m^2  min_area=1e-20 in^2  max_area=(pi*(pipe_HD-0.0001)^2)/4 in^2  area=(pi*pipe_HD^2)/4 in^2  Cd=0.64  B_lam=0.999
      settings: SourceProductBaseCode=PW,SS,VE
  PS Constant1 : fl_lib/Physical Signals/Sources/PS Constant  constant=0.21
      settings: SourceProductBaseCode=PW,SS,VE
  PS Constant2 : fl_lib/Physical Signals/Sources/PS Constant  constant=room_temp K
      settings: SourceProductBaseCode=PW,SS,VE
  PS Constant3 : fl_lib/Physical Signals/Sources/PS Constant  constant=room_pressure*6895.76 Pa
      settings: SourceProductBaseCode=PW,SS,VE
  PS Switch2 : fl_lib/Physical Signals/Nonlinear Operators/PS Switch  Threshold=1
      settings: SourceProductBaseCode=PW,SS,VE  InternalSimscapePortConfiguration="{\"Bottom\":[],\"Left\":[{\"id\":\"I1\",\"label\":\"\",\"type\":\"input\"},{\"id\":\"I2\",\"label\":\"\",\"type\":\"input\"},{\"id\":\"I3\",\"label\":\"\",\"type\":\"input\"}],\"Right\":[{\"id\":\"O\",\"label\":\"\",\"type\":\"output\"}],\"Top\":[]}"
  Simulink-PS Converter3 : nesl_utility/Simulink-PS Converter  PhysicalDomain=network_engine_domain  SubClassName=ps_input  LeftPortType=input  RightPortType=output  PseudoPeriodic=off  Frequencies=[]  NoiseDistribution=none  NoiseParameters=[]  Unit=Pa  AffineConversion=off  FilteringAndDerivatives=provide  SimscapeFilterOrder=1  InputFilterTimeConstant=0.001  UdotUserProvided=0
      settings: SourceProductBaseCode=SS,PW,VE
  Simulink-PS Converter4 : nesl_utility/Simulink-PS Converter  PhysicalDomain=network_engine_domain  SubClassName=ps_input  LeftPortType=input  RightPortType=output  PseudoPeriodic=off  Frequencies=[]  NoiseDistribution=none  NoiseParameters=[]  Unit=Pa  AffineConversion=off  FilteringAndDerivatives=provide  SimscapeFilterOrder=1  InputFilterTimeConstant=0.001  UdotUserProvided=0
      settings: SourceProductBaseCode=SS,PW,VE
  input : PMIOPort  Side=Left
  Conn2 : PMIOPort  Port=2  Side=Right
  sig : PMIOPort  Port=3  Side=Left
  wires:
  Constant3/1 -> Simulink-PS Converter3/1
  Constant4/1 -> Simulink-PS Converter4/1
  connections:
  input/RConn1 -- Local Restriction (MA)1/LConn2
  Controlled Reservoir (MA)/LConn1 -- Local Restriction (MA)1/LConn1
  PS Constant3/RConn1 -- Controlled Reservoir (MA)/RConn2
  Lab CO2 concentration NOT inlet CO2/RConn1 -- Controlled Reservoir (MA)/RConn4
  PS Constant1/RConn1 -- Controlled Reservoir (MA)/RConn3
  PS Constant2/RConn1 -- Controlled Reservoir (MA)/RConn1
  Simulink-PS Converter4/RConn1 -- PS Switch2/LConn1
  Simulink-PS Converter3/RConn1 -- PS Switch2/LConn3
  Controlled Pressure Source (MA)/LConn1 -- Local Restriction (MA)1/RConn1
  Controlled Pressure Source (MA)/RConn1 -- Conn2/RConn1
  PS Switch2/RConn1 -- Controlled Pressure Source (MA)/LConn2
  sig/RConn1 -- PS Switch2/LConn2

== system STEVE_ver28/Selector Valve ==
  Local Restriction (MA)1 : fl_lib/Moist Air/Elements/Local Restriction (MA)  restriction_type=foundation.enum.restriction_type.variable  restriction_area=0.001 m^2  min_area=1e-20 in^2  max_area=(pi*(pipe_HD-0.0001)^2)/4 in^2  area=(pi*pipe_HD^2)/4 in^2  Cd=0.64  B_lam=0.999
      settings: SourceProductBaseCode=PW,SS,VE
  In : PMIOPort  Side=Left
  Flow Out : PMIOPort  Port=2  Side=Right
  Command : PMIOPort  Port=3  Side=Left
  Vac Out : PMIOPort  Port=4  Side=Right
  connections:
  Flow Out/RConn1 -- Vac Out/RConn1 -- Local Restriction (MA)1/RConn1
  Local Restriction (MA)1/LConn1 -- In/RConn1
  Local Restriction (MA)1/LConn2 -- Command/RConn1
